simulink model "Q2_sim"  (R2021a)
settings: Solver=VariableStepAuto  StartTime=0.0  StopTime=30  RelTol=1e-3
values from neighbouring files (symbols this model uses):
  A = [-1.7,-0.25,0;23,-30,20;0,-200-290,-220-920]    [Q1_code.m]    (also in Q2_code.m; Q3_code.m; Q4_code.m; Q5_code.m)
  B = [3+2,0;-30-53,0;0,-420-350]    [Q1_code.m]    (also in Q2_code.m; Q3_code.m; Q4_code.m; Q5_code.m)
  C1 = eye(3)    [Q2_code.m]    (also in Q3_code.m; Q4_code.m)
  D1 = zeros(3,2)    [Q2_code.m]    (also in Q3_code.m; Q4_code.m)
  x0 = [1;100;200]    [Q2_code.m]    (also in Q3_code.m; Q4_code.m; Q5_code.m; Q6_code.m)
undefined symbols (not defined in the file or in its folder): Kr
settings Model: Creator=l_w_h  LastModifiedBy=l_w_h

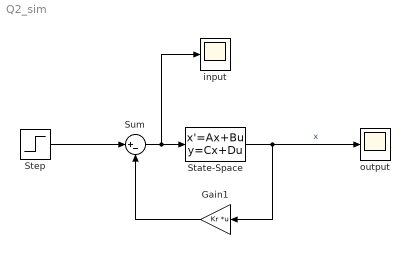
== system Q2_sim ==
  Gain1 : Gain  Gain=Kr  Multiplication=Matrix(K*u)
  State-Space : StateSpace  A=A  B=B  C=C1  D=D1  InitialCondition=x0
  Step : Step  Time=0  After=[0;0]  SampleTime=0
  Sum : Sum  Inputs=|+-
  input : Scope
  output : Scope
  wires:
  State-Space/1 -> output/1, Gain1/1  "x"
  Gain1/1 -> Sum/2
  Sum/1 -> input/1, State-Space/1
  Step/1 -> Sum/1
